simulink model "test_PassVeh_acc"  (R2018b)
settings: configuration reference "Physics" (kept outside this file)
model workspace (MAT data in the model file):
  m = 1000
libraries: simulink x1
settings Model: DataDictionary=test_PassengerVehicle.sldd  PauseTimes=9.280  Creator=wischnewski  LastModifiedBy=Michael

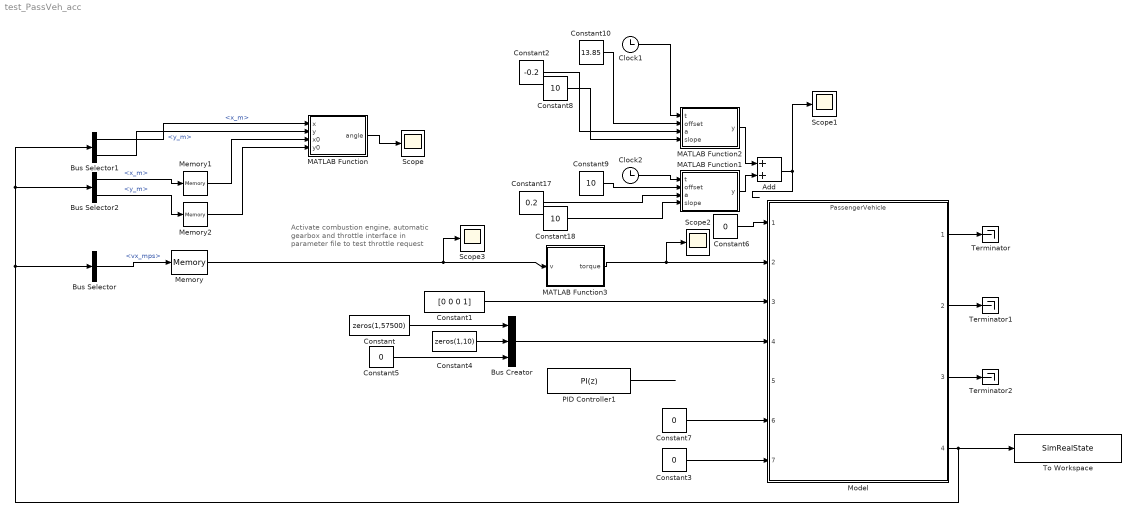
== system test_PassVeh_acc ==
  note: Activate combustion engine, automatic gearbox and throttle interface in parameter file to test throttle request
  Add : Sum
  Bus Creator : BusCreator  Inputs=3  OutDataTypeStr=Bus: tpamapReference
  Bus Selector : BusSelector  OutputSignals=vx_mps
  Bus Selector1 : BusSelector  OutputSignals=x_m,y_m
  Bus Selector2 : BusSelector  OutputSignals=x_m,y_m
  Clock1 : Clock
  Clock2 : Clock
  Constant : Constant  Value=zeros(1,57500)
  Constant1 : Constant  Value=[0 0 0 1]
  Constant10 : Constant  Value=13.85
  Constant17 : Constant  Value=0.2
  Constant18 : Constant  Value=10
  Constant2 : Constant  Value=-0.2
  Constant{3,5..7} (4 alike) : Constant  Value=0
  Constant4 : Constant  Value=zeros(1,10)
  Constant8 : Constant  Value=10
  Constant9 : Constant  Value=10
  MATLAB Function : MATLAB Function  TreatAsAtomicUnit=on
  MATLAB Function1 : MATLAB Function  TreatAsAtomicUnit=on
  MATLAB Function2 : MATLAB Function  TreatAsAtomicUnit=on
  MATLAB Function3 : MATLAB Function  TreatAsAtomicUnit=on
  Memory : Memory
  Memory1 : Memory
  Memory2 : Memory
  Model : ModelReference  ModelNameDialog=PassengerVehicle.slx  SimulationMode=Normal  ModelReferenceVersion=1.935
  PID Controller1 : simulink/Continuous/PID Controller  Controller=PI  Form=Parallel  TimeDomain=Discrete-time  SampleTime=-1  IntegratorMethod=Forward Euler  FilterMethod=Forward Euler  ControllerParametersSource=internal  P=1  I=0.1  D=0  UseFilter=on  N=100  TunerSelectOption=Transfer Function Based (PID Tuner App)  InitialConditionSource=internal  InitialConditionForIntegrator=0  InitialConditionForFilter=0  DifferentiatorICPrevScaledInput=0  ExternalReset=none  TrackingMode=off  Kt=1  LimitOutput=on  UpperSaturationLimit=1  LowerSaturationLimit=0  LinearizeAsGain=on  AntiWindupMode=none  Kb=1  POutMin=[]  POutMax=[]  IOutMin=[]  IOutMax=[]  DOutMin=[]  DOutMax=[]  NOutMin=[]  NOutMax=[]  SumOutMin=[]  SumOutMax=[]  SaturationOutMin=[]  SaturationOutMax=[]  PParamMin=[]  PParamMax=[]  IParamMin=[]  IParamMax=[]  DParamMin=[]  DParamMax=[]  NParamMin=[]  NParamMax=[]  KbParamMin=[]  KbParamMax=[]  KtParamMin=[]  KtParamMax=[]  KbOutMin=[]  KbOutMax=[]  KtOutMin=[]  KtOutMax=[]  IntegratorOutMin=[]  IntegratorOutMax=[]  FilterOutMin=[]  FilterOutMax=[]  SumI1OutMin=[]  SumI1OutMax=[]  SumI2OutMin=[]  SumI2OutMax=[]  SumI3OutMin=[]  SumI3OutMax=[]  SumI4OutMin=[]  SumI4OutMax=[]  SumDOutMin=[]  SumDOutMax=[]  DifferentiatorOutMin=[]  DifferentiatorOutMax=[]  FilterDiffOutCoefMin=[]  FilterDiffOutCoefMax=[]  ReciprocalOutMin=[]  ReciprocalOutMax=[]  SumDenOutMin=[]  SumDenOutMax=[]  SumNumOutMin=[]  SumNumOutMax=[]  DivideOutMin=[]  DivideOutMax=[]  IntegratorContinuousStateAttributes=''  IntegratorStateMustResolveToSignalObject=off  IntegratorRTWStateStorageClass=Auto  FilterContinuousStateAttributes=''  FilterStateMustResolveToSignalObject=off  FilterRTWStateStorageClass=Auto  ParallelPVariant=InternalParameters  IdealPVariant=Disabled  IVariant=InternalParameters  DVariant=Disabled  IntegratorVariant=Discrete  SatVariant=Enabled  AWVariant=Passthrough  PCopyVariant=Disabled  TRVariant=Disabled  FdbkBlocksVariant=Forward  IdealPFdbkVariant=Disabled  SatFdbkVariant=Disabled  DerivativeFilterVariant=Disabled  NVariant=Disabled  NCopyVariant=Disabled_SignalSpec  FilterICVariant=Disabled  IntegratorICVariant=InternalICs  ExternalResetVariant=Disabled  TRSumVariant=Passthrough  SumFdbkVariant=Disabled  SumVariant=Sum_PI
  Scope{,1..3} (4 alike) : Scope
  Terminator : Terminator
  Terminator1 : Terminator
  Terminator2 : Terminator
  To Workspace : ToWorkspace  VariableName=SimRealState  SaveFormat=Timeseries  SampleTime=-1
  wires:
  Bus Creator/1 -> Model/4
  Constant1/1 -> Model/3
  Model/1 -> Terminator/1
  Model/3 -> Terminator2/1
  Model/2 -> Terminator1/1
  Constant/1 -> Bus Creator/1
  Constant4/1 -> Bus Creator/2
  Constant5/1 -> Bus Creator/3
  Model/4 -> To Workspace/1, Bus Selector2/1, Bus Selector1/1, Bus Selector/1
  Bus Selector/1 -> Memory/1  "<vx_mps>"
  Memory/1 -> Scope3/1, MATLAB Function3/1(v)
  Constant7/1 -> Model/6
  Constant3/1 -> Model/7
  PID Controller1/1 -> ?
  Bus Selector1/1 -> MATLAB Function/1(x)  "<x_m>"
  Bus Selector1/2 -> MATLAB Function/2(y)  "<y_m>"
  Bus Selector2/1 -> Memory1/1  "<x_m>"
  Bus Selector2/2 -> Memory2/1  "<y_m>"
  Memory2/1 -> MATLAB Function/4(y0)
  Memory1/1 -> MATLAB Function/3(x0)
  Clock2/1 -> MATLAB Function1/1(t)
  Constant9/1 -> MATLAB Function1/2(offset)
  Constant17/1 -> MATLAB Function1/3(a)
  Constant18/1 -> MATLAB Function1/4(slope)
  MATLAB Function1/1(y) -> Add/2
  Clock1/1 -> MATLAB Function2/1(t)
  Constant10/1 -> MATLAB Function2/2(offset)
  Constant2/1 -> MATLAB Function2/3(a)
  Constant8/1 -> MATLAB Function2/4(slope)
  MATLAB Function2/1(y) -> Add/1
  Add/1 -> Scope1/1
  MATLAB Function/1(angle) -> Scope/1
  MATLAB Function3/1(torque) -> Scope2/1, Model/2
  Constant6/1 -> Model/1

== matlab function test_PassVeh_acc/MATLAB Function1 ==
  data: t input; y output; offset input; a input; slope input
function y = sigmoid(t, offset, a, slope)

y = a/(1+exp(-slope*(t-offset)));

end

== matlab function test_PassVeh_acc/MATLAB Function ==
  data: x input; angle output; y input; x0 input; y0 input
function angle=rotationIndex(x, y, x0, y0)

    xVec = x-x0;
    yVec = y-y0;

    angle = atan(yVec/xVec);
    
    if xVec >= 0 && yVec >= 0
        return;
        
    elseif xVec >= 0 && yVec <= 0 
        angle = angle + 2*pi();
        
    else
        angle = angle + pi(); 
    end

return;
end

== matlab function test_PassVeh_acc/MATLAB Function2 ==
  data: t input; y output; offset input; a input; slope input
function y = sigmoid(t, offset, a, slope)

y = a/(1+exp(-slope*(t-offset)));

end

== matlab function test_PassVeh_acc/MATLAB Function3 ==
  data: v input; torque output
function torque = torqueFromRPM(v)

% uses indexing to return the corresponding torque from the closest RPM
% value to the input velocity

motorCurve = [	50.66205277	, 	230.2197308	;
	157.9218215	, 	230.2197308	;
	265.1815902	, 	230.2197308	;
	372.441359	, 	230.2197308	;
	479.7011277	, 	230.2197308	;
	586.9608964	, 	230.2197308	;
	694.2206651	, 	230.2197308	;
	801.7851491	, 	230.3330272	;
	908.7402026	, 	230.2197308	;
	1015.999971	, 	230.2197308	;
	1123.25974	, 	230.2197308	;
	1230.519509	, 	230.2197308	;
	1331.075542	, 	230.2197308	;
	1438.335311	, 	230.2197308	;
	1545.595079	, 	230.2197308	;
	1652.854848	, 	230.2197308	;
	1760.114617	, 	230.2197308	;
	1867.374386	, 	230.2197308	;
	1974.634154	, 	230.2197308	;
	2081.893923	, 	230.2197308	;
	2189.153692	, 	230.2197308	;
	2296.413461	, 	230.2197308	;
	2403.368514	, 	230.3330272	;
	2510.932998	, 	230.2197308	;
	2612.60632	, 	230.158187	;
	2720.759921	, 	230.0812574	;
	2826.008569	, 	229.942784	;
	2933.268337	, 	228.2642088	;
	3040.528106	, 	220.2776953	;
	3140.087902	, 	213.3376885	;
	3210.749726	, 	208.6552417	;
	3309.794817	, 	202.4236054	;
	3415.937297	, 	196.1865995	;
	3523.197065	, 	190.2705113	;
	3630.456834	, 	184.641364	;
	3737.716603	, 	179.3424494	;
	3844.976372	, 	174.3909126	;
	3945.532405	, 	169.9386644	;
	4053.706319	, 	165.4507095	;
	4160.051942	, 	161.230621	;
	4267.311711	, 	157.2236064	;
	4374.57148	, 	153.4607535	;
	4480.917103	, 	149.9403181	;
	4589.091017	, 	146.6016031	;
	4694.339665	, 	143.5183743	;
	4801.477548	, 	140.5572875	;
	4907.518455	, 	137.7911831	;
	5014.778224	, 	135.0915126	;
	5122.037993	, 	132.5076581	;
	5227.957015	, 	130.047608	;
	5326.501927	, 	127.9358716	;
	5433.456981	, 	125.6093481	];

% wheel radius
r = 0.21;

% separating torque and RPM lists from motor curves
torqueList = motorCurve(:,2)*4/r;
rpmList = motorCurve(:,1);
len = length(rpmList);

% converting v (m/s) to rpm
rpm = 60*v*2/(pi()*r);

index = 1; 
minDiff = 10000;

for i = 1:len
    diff = abs(rpmList(i) - rpm);
    if diff < minDiff
        minDiff = diff;
        index = i;
    end
end

torque = torqueList(index);

end
